simulink model "inverted_pendulum"  (R2018b)
settings: Solver=VariableStepAuto  StartTime=0.0  StopTime=20  RelTol=1e-3
undefined symbols (not defined in the file): g, Kd, Kp, L
settings Model: Creator=sergeyroyz  LastModifiedBy=sergeyroyz

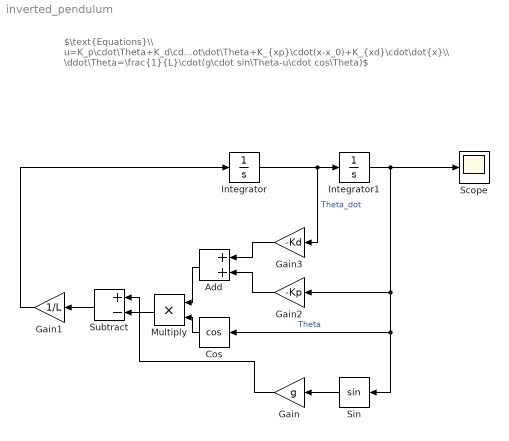
== system inverted_pendulum ==
  note: $\text{Equations}\\ u=K_p\cdot\Theta+K_d\cdot\dot\Theta+K_{xp}\cdot(x-x_0)+K_{xd}\cdot\dot{x}\\ \ddot\Theta=\frac{1}{L}\cdot(g\cdot sin\Theta-u\cdot cos\Theta)$
  Add : Sum
  Cos : Trigonometry  Operator=cos
  Gain : Gain  Gain=g
  Gain1 : Gain  Gain=1/L
  Gain2 : Gain  Gain=-Kp
  Gain3 : Gain  Gain=-Kd
  Integrator : Integrator  InitialCondition=0.01
  Integrator1 : Integrator
  Multiply : Product
  Scope : Scope
  Sin : Trigonometry
  Subtract : Sum  Inputs=+-
  wires:
  Integrator/1 -> Gain3/1, Integrator1/1  "Theta_dot"
  Gain1/1 -> Integrator/1
  Integrator1/1 -> Gain2/1, Cos/1, Sin/1, Scope/1  "Theta"
  Sin/1 -> Gain/1
  Gain2/1 -> Add/2
  Gain3/1 -> Add/1
  Add/1 -> Multiply/1
  Cos/1 -> Multiply/2
  Gain/1 -> Subtract/1
  Multiply/1 -> Subtract/2
  Subtract/1 -> Gain1/1
